simulink model "sumtime_example"  (Simulink 7.6)
settings: Solver=ode45  StartTime=0.0  StopTime=24*3600+1  RelTol=1e-3
libraries: carnot x2
settings Model: Creator=drhf  LastModifiedBy=drhf

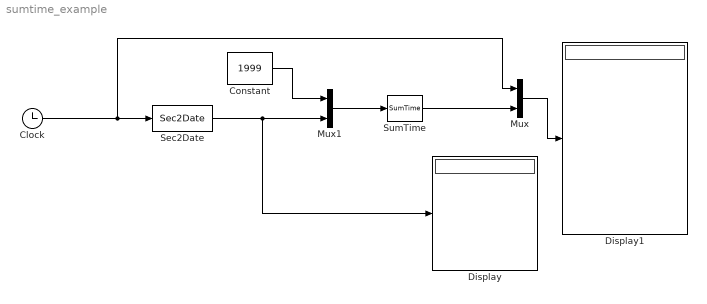
== system sumtime_example ==
  Clock : Clock
      settings: Decimation=10
  Constant : Constant  Value=1999
  Display : Display
  Display1 : Display
  Mux : Mux  Inputs=2
  Mux1 : Mux  Inputs=2
  Sec2Date : carnot/Toolbox/Sec2Date
  SumTime : carnot/Toolbox/SumTime
  wires:
  Sec2Date/1 -> Display/1, Mux1/2
  Clock/1 -> Sec2Date/1, Mux/1
  Mux/1 -> Display1/1
  Mux1/1 -> SumTime/1
  Constant/1 -> Mux1/1
  SumTime/1 -> Mux/2
